simulink model "AbabilFlightController_Android"  (R2021a)
settings: Solver=ode3  StartTime=0.0  StopTime=40.0  RelTol=1e-3
InitFcn:
  | Ts=0.01
  | kFactor = 1.2;
  | 
  | KpRollAttitude = 0.630138625117681 / kFactor;
  | KiRollAttitude = 0.0552303199591522 / kFactor;
  | 
  | KpPitchAttitude = 0.630138625117681 / kFactor;
  | KiPitchAttitude = 0.0552303199591522 / kFactor;
  | 
  | KpRollRate = 1.31533836563383 / kFactor;
  | KiRollRate = 0.460338699849681 / kFactor;
  | 
  | KpPitchRate = 1.31533836563383 / kFactor;
  | KiPitchRate = 0.460338699849681 / kFactor;
  | 
  | KpYawRate = 1.31533836563383 / kFactor;
  | KiYawRate = 0.460338699849681 / kFactor;
undefined symbols (not defined in the file): Accel, AHRS_Ang_Vel, AHRS_Attitude, Alt, androidSerialSendReceive, AttiudeFiltered, Data_Input, fdesignblkfcn, gcbh, Gyro, kalman, Mag, Static_Orientation
libraries: androiduilib x10, androidsensorlib x5, pid_lib x5, androidcommunicationlib x2, mspfiltlib x1, simulink_extras x1, simulink x1, aerolibatmos2 x1
(part 1 of 2)
PreSaveFcn:
  | set_param(gcs, 'Location',[35 56 895 605])
settings Model: ExtModeTrigDuration=100  Creator=The MathWorks, Inc.  LastModifiedBy=AA
settings SolverCC: AlgebraicLoopSolver=TrustRegion
settings DataIOCC: LimitDataPoints=on  SaveFormat=Array  ReturnWorkspaceOutputs=off
settings OptimizationCC: LifeSpan=1  MaxStackSize=64
settings DebuggingCC: UnderspecifiedInitializationDetection=Classic  MergeDetectMultiDrivingBlocksExec=none  ParameterPrecisionLossMsg=none  AllowSymbolicDim=off  SFUnexpectedBacktrackingDiag=warning  SFNoUnconditionalDefaultTransitionDiag=warning  SFExecutionAtInitializationDiag=none  SFMachineParentedDataDiag=warning  ArithmeticOperatorsInVariantConditions=warning
settings HardwareCC: ProdBitPerPointer=32  ProdBitPerSizeT=32  ProdBitPerPtrDiffT=32  ProdLargestAtomicInteger=Long  ProdLargestAtomicFloat=Double  ProdWordSize=32  ProdHWDeviceType=ARM Compatible->ARM Cortex  TargetLargestAtomicInteger=Long  TargetLargestAtomicFloat=Double  TargetEndianess=LittleEndian  TargetHWDeviceType=ARM Compatible->ARM Cortex  UseEmbeddedCoderFeatures=off  UseSimulinkCoderFeatures=off
settings ModelReferenceCC: PropagateSignalLabelsOutOfModel=off
settings SFSimCC: SimUseLocalCustomCode=off  CustomCodeUndefinedFunction=UseInterfaceOnly
settings RTWCC: SystemTargetFile=ert.tlc  HardwareBoard=Android Device  TemplateMakefile=ert_default_tmf  GenerateReport=on  RTWVerbose=off  RTWUseLocalCustomCode=off  Toolchain=Android SDK/NDK Tools  LaunchReport=on
settings CodeAppCC: ForceParamTrailComments=on  OperatorAnnotations=on  StateflowObjectComments=on  MATLABSourceComments=on
settings ERTTargetCC: MultiwordLength=2048  ERTCustomFileBanners=off  SupportContinuousTime=on  SupportNonInlinedSFcns=on  RemoveResetFunc=off  ModelStepFunctionPrototypeControlCompliant=off
settings ConfigComp: CovMetricSettings=dw  CovSaveCumulativeToWorkspaceVar=on  CovSaveSingleToWorkspaceVar=on  CovExternalEMLEnable=off  CovSFcnEnable=off

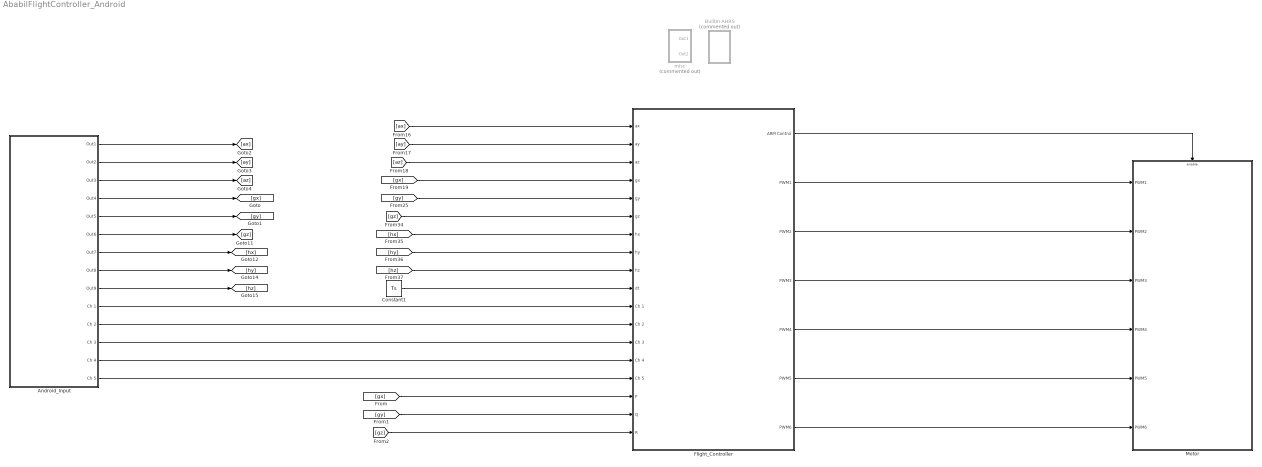
== system AbabilFlightController_Android ==
  Android_Input : Subsystem
  BuiltIn AHRS : Subsystem  Commented=on
  Constant1 : Constant  Value=Ts
  Flight_Controller : Subsystem
  Motor : Subsystem  TreatAsAtomicUnit=on
  misc : Subsystem  Commented=on
  wires:
  Android_Input/3(Out3) -> [az]
  Android_Input/6(Out6) -> [gz]
  [ax] -> Flight_Controller/1(ax)
  [ay] -> Flight_Controller/2(ay)
  [az] -> Flight_Controller/3(az)
  [gy] -> Flight_Controller/5(gy)
  [gx] -> Flight_Controller/4(gx)
  [gz] -> Flight_Controller/6(gz)
  [hz] -> Flight_Controller/9(hz)
  [hy] -> Flight_Controller/8(hy)
  [hx] -> Flight_Controller/7(hx)
  Constant1/1 -> Flight_Controller/10(dt)
  Android_Input/1(Out1) -> [ax]
  Android_Input/2(Out2) -> [ay]
  Android_Input/4(Out4) -> [gx]
  Android_Input/5(Out5) -> [gy]
  Android_Input/7(Out7) -> [hx]
  Android_Input/8(Out8) -> [hy]
  Android_Input/9(Out9) -> [hz]
  [gy] -> Flight_Controller/17(Q)
  [gx] -> Flight_Controller/16(P)
  [gz] -> Flight_Controller/18(R)
  Android_Input/10(Ch 1) -> Flight_Controller/11(Ch 1)
  Android_Input/11(Ch 2) -> Flight_Controller/12(Ch 2)
  Android_Input/12(Ch 3) -> Flight_Controller/13(Ch 3)
  Android_Input/13(Ch 4) -> Flight_Controller/14(Ch 4)
  Android_Input/14(Ch 5) -> Flight_Controller/15(Ch 5)
  Flight_Controller/2(PWM1) -> Motor/1(PWM1)
  Flight_Controller/3(PWM2) -> Motor/2(PWM2)
  Flight_Controller/4(PWM3) -> Motor/3(PWM3)
  Flight_Controller/5(PWM4) -> Motor/4(PWM4)
  Flight_Controller/6(PWM5) -> Motor/5(PWM5)
  Flight_Controller/7(PWM6) -> Motor/6(PWM6)
  Flight_Controller/1(ARM Control) -> Motor/Enable

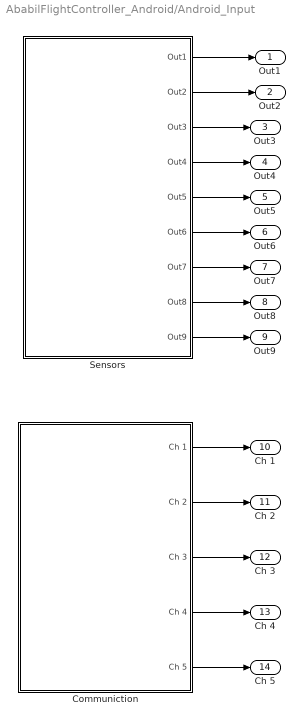
== system AbabilFlightController_Android/Android_Input ==
  Communiction : Subsystem
  Sensors : Subsystem
  Out1 : Outport
  Out2 : Outport  Port=2
  Out3 : Outport  Port=3
  Out4 : Outport  Port=4
  Out5 : Outport  Port=5
  Out6 : Outport  Port=6
  Out7 : Outport  Port=7
  Out8 : Outport  Port=8
  Out9 : Outport  Port=9
  Ch 1 : Outport  Port=10
  Ch 2 : Outport  Port=11
  Ch 3 : Outport  Port=12
  Ch 4 : Outport  Port=13
  Ch 5 : Outport  Port=14
  wires:
  Sensors/1(Out1) -> Out1/1
  Sensors/2(Out2) -> Out2/1
  Sensors/3(Out3) -> Out3/1
  Sensors/4(Out4) -> Out4/1
  Sensors/5(Out5) -> Out5/1
  Sensors/6(Out6) -> Out6/1
  Sensors/7(Out7) -> Out7/1
  Sensors/8(Out8) -> Out8/1
  Sensors/9(Out9) -> Out9/1
  Communiction/1(Ch 1) -> Ch 1/1
  Communiction/2(Ch 2) -> Ch 2/1
  Communiction/3(Ch 3) -> Ch 3/1
  Communiction/4(Ch 4) -> Ch 4/1
  Communiction/5(Ch 5) -> Ch 5/1

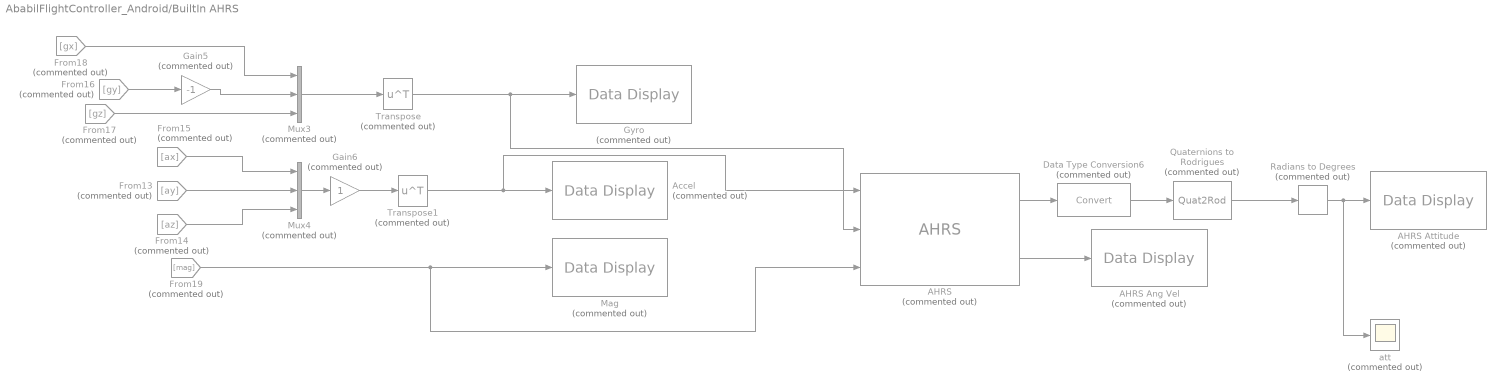
== system AbabilFlightController_Android/BuiltIn AHRS ==
  AHRS : mspfiltlib/AHRS  Commented=on  DispRefFrame=NED  DecimationFactor=1  InitialProcessNoise=ahrsfilter.defaultProcessNoise  OrientationFormat=quaternion  SimulateUsing=Code generation  AccelerometerNoise=7.7792e-07  GyroscopeNoise=3.7046e-08  MagnetometerNoise=0.1  GyroscopeDriftNoise=3.0462e-13  LinearAccelerationNoise=0.0096236100000000012  MagneticDisturbanceNoise=0.5  LinearAccelerationDecayFactor=0.5  MagneticDisturbanceDecayFactor=0.5  ExpectedMagneticFieldStrength=50
      settings: SourceProductBaseCode=TF,NV
  AHRS Ang Vel : androiduilib/Data Display  Commented=on  DataDisplayId=kalman/AHRS_Ang_Vel  Format=Float  Precision=6  SimulateUsing=Code generation  blockPlatform=Android
      settings: SourceProductBaseCode=ANDROID
  AHRS Attitude : androiduilib/Data Display  Commented=on  DataDisplayId=kalman/AHRS_Attitude  Format=Float  Precision=6  SimulateUsing=Code generation  blockPlatform=Android
      settings: SourceProductBaseCode=ANDROID
  Accel : androiduilib/Data Display  Commented=on  DataDisplayId=kalman/Accel  Format=Float  Precision=6  SimulateUsing=Code generation  blockPlatform=Android
      settings: SourceProductBaseCode=ANDROID
  Data Type Conversion6 : DataTypeConversion  Commented=on
  From13 : From  Commented=on  GotoTag=ay
  From14 : From  Commented=on  GotoTag=az
  From15 : From  Commented=on  GotoTag=ax
  From16 : From  Commented=on  GotoTag=gy
  From17 : From  Commented=on  GotoTag=gz
  From18 : From  Commented=on  GotoTag=gx
  From19 : From  Commented=on  GotoTag=mag
  Gain5 : Gain  Commented=on  Gain=-1
  Gain6 : Gain  Commented=on
  Gyro : androiduilib/Data Display  Commented=on  DataDisplayId=kalman/Gyro  Format=Float  Precision=6  SimulateUsing=Code generation  blockPlatform=Android
      settings: SourceProductBaseCode=ANDROID
  Mag : androiduilib/Data Display  Commented=on  DataDisplayId=kalman/Mag  Format=Float  Precision=6  SimulateUsing=Code generation  blockPlatform=Android
      settings: SourceProductBaseCode=ANDROID
  Mux3 : Mux  Commented=on  Inputs=3
  Mux4 : Mux  Commented=on  Inputs=3
  Quaternions to Rodrigues : Quat2Rod  Commented=on
  Radians to Degrees : simulink_extras/Transformations/Radians to Degrees  Commented=on
  Transpose : Math  Commented=on  Operator=transpose  SaturateOnIntegerOverflow=on
  Transpose1 : Math  Commented=on  Operator=transpose  SaturateOnIntegerOverflow=on
  att : Scope  Commented=on
  wires:
  From18/1 -> Mux3/1
  From14/1 -> Mux4/3
  AHRS/2 -> AHRS Ang Vel/1
  Transpose/1 -> AHRS/2, Gyro/1
  From17/1 -> Mux3/3
  Mux4/1 -> Gain6/1
  Transpose1/1 -> AHRS/1, Accel/1
  From15/1 -> Mux4/1
  From19/1 -> AHRS/3, Mag/1
  From13/1 -> Mux4/2
  AHRS/1 -> Data Type Conversion6/1
  Data Type Conversion6/1 -> Quaternions to Rodrigues/1
  Quaternions to Rodrigues/1 -> Radians to Degrees/1
  Radians to Degrees/1 -> att/1, AHRS Attitude/1
  Gain6/1 -> Transpose1/1
  Gain5/1 -> Mux3/2
  From16/1 -> Gain5/1
  Mux3/1 -> Transpose/1

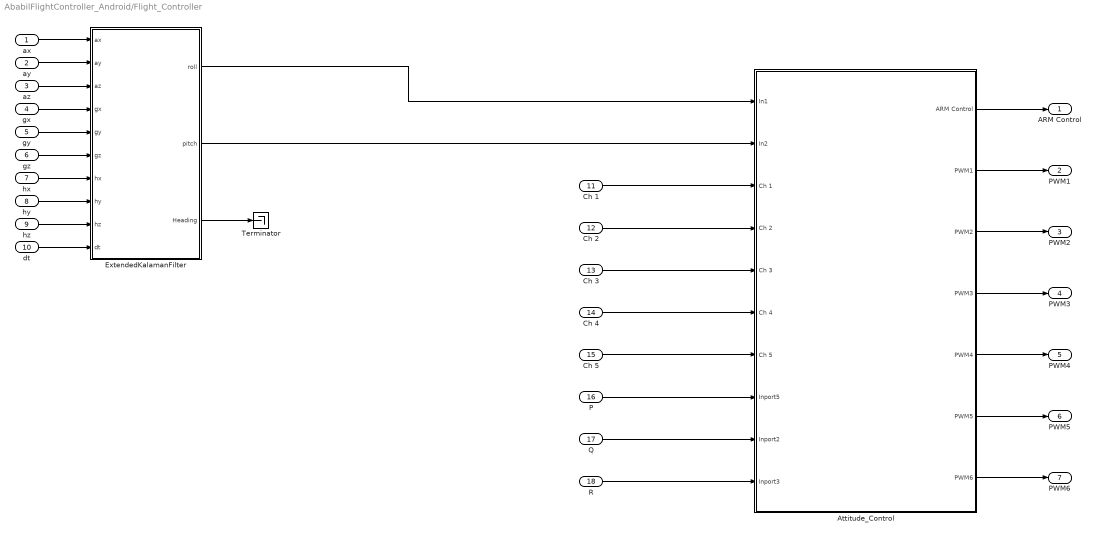
== system AbabilFlightController_Android/Flight_Controller ==
  ax : Inport
  ay : Inport  Port=2
  az : Inport  Port=3
  gx : Inport  Port=4
  gy : Inport  Port=5
  gz : Inport  Port=6
  hx : Inport  Port=7
  hy : Inport  Port=8
  hz : Inport  Port=9
  dt : Inport  Port=10
  Ch 1 : Inport  Port=11
  Ch 2 : Inport  Port=12
  Ch 3 : Inport  Port=13
  Ch 4 : Inport  Port=14
  Ch 5 : Inport  Port=15
  P : Inport  Port=16
  Q : Inport  Port=17
  R : Inport  Port=18
  Attitude_Control : Subsystem
  ExtendedKalamanFilter : Subsystem
  Terminator : Terminator
  ARM Control : Outport
  PWM1 : Outport  Port=2
  PWM2 : Outport  Port=3
  PWM3 : Outport  Port=4
  PWM4 : Outport  Port=5
  PWM5 : Outport  Port=6
  PWM6 : Outport  Port=7
  wires:
  ExtendedKalamanFilter/2(pitch) -> Attitude_Control/2(In2)
  ExtendedKalamanFilter/1(roll) -> Attitude_Control/1(In1)
  ExtendedKalamanFilter/3(Heading) -> Terminator/1
  ax/1 -> ExtendedKalamanFilter/1(ax)
  ay/1 -> ExtendedKalamanFilter/2(ay)
  az/1 -> ExtendedKalamanFilter/3(az)
  gx/1 -> ExtendedKalamanFilter/4(gx)
  gy/1 -> ExtendedKalamanFilter/5(gy)
  gz/1 -> ExtendedKalamanFilter/6(gz)
  hx/1 -> ExtendedKalamanFilter/7(hx)
  hy/1 -> ExtendedKalamanFilter/8(hy)
  hz/1 -> ExtendedKalamanFilter/9(hz)
  dt/1 -> ExtendedKalamanFilter/10(dt)
  Attitude_Control/7(PWM6) -> PWM6/1
  Attitude_Control/6(PWM5) -> PWM5/1
  Attitude_Control/5(PWM4) -> PWM4/1
  Attitude_Control/4(PWM3) -> PWM3/1
  Attitude_Control/3(PWM2) -> PWM2/1
  Attitude_Control/2(PWM1) -> PWM1/1
  Attitude_Control/1(ARM Control) -> ARM Control/1
  Ch 1/1 -> Attitude_Control/3(Ch 1)
  Ch 2/1 -> Attitude_Control/4(Ch 2)
  Ch 3/1 -> Attitude_Control/5(Ch 3)
  Ch 4/1 -> Attitude_Control/6(Ch 4)
  Ch 5/1 -> Attitude_Control/7(Ch 5)
  P/1 -> Attitude_Control/8(Inport5)
  Q/1 -> Attitude_Control/9(Inport2)
  R/1 -> Attitude_Control/10(Inport3)

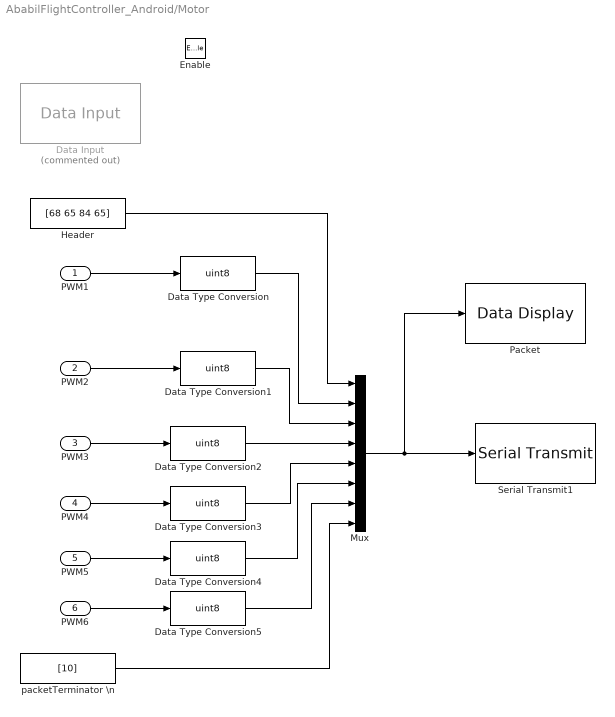
== system AbabilFlightController_Android/Motor ==
  PWM1 : Inport
  PWM2 : Inport  Port=2
  PWM3 : Inport  Port=3
  PWM4 : Inport  Port=4
  PWM5 : Inport  Port=5
  PWM6 : Inport  Port=6
  Enable : EnablePort
  Data Input : androiduilib/Data Input  Commented=on  isCharVector=on  Value=1.0  CharVector=DATA  OutputDataType=double  maxCharVectorSize=4  DataInputId=androidSerialSendReceive/Data_Input  SampleTime=Ts
      settings: SourceProductBaseCode=ANDROID
  Data Type Conversion{,1..5} (6 alike) : DataTypeConversion  OutDataTypeStr=uint8
  Header : Constant  Value=[68 65 84 65]  OutDataTypeStr=uint8  SampleTime=Ts
  Mux : Mux  Inputs=8
  Packet : androiduilib/Data Display  DataDisplayId=Ababil/Motor/Packet  Format=Integer  Precision=6  SimulateUsing=Code generation  blockPlatform=Android
      settings: SourceProductBaseCode=ANDROID
  Serial Transmit1 : androidcommunicationlib/Serial Transmit
      settings: SourceProductBaseCode=ANDROID
  packetTerminator \n : Constant  Value=[10]  OutDataTypeStr=uint8
  wires:
  PWM1/1 -> Data Type Conversion/1
  PWM5/1 -> Data Type Conversion4/1
  PWM2/1 -> Data Type Conversion1/1
  PWM6/1 -> Data Type Conversion5/1
  PWM4/1 -> Data Type Conversion3/1
  Data Type Conversion2/1 -> Mux/4
  Data Type Conversion3/1 -> Mux/5
  Data Type Conversion/1 -> Mux/2
  PWM3/1 -> Data Type Conversion2/1
  Data Type Conversion4/1 -> Mux/6
  Mux/1 -> Packet/1, Serial Transmit1/1
  Data Type Conversion5/1 -> Mux/7
  packetTerminator \n/1 -> Mux/8
  Header/1 -> Mux/1
  Data Type Conversion1/1 -> Mux/3

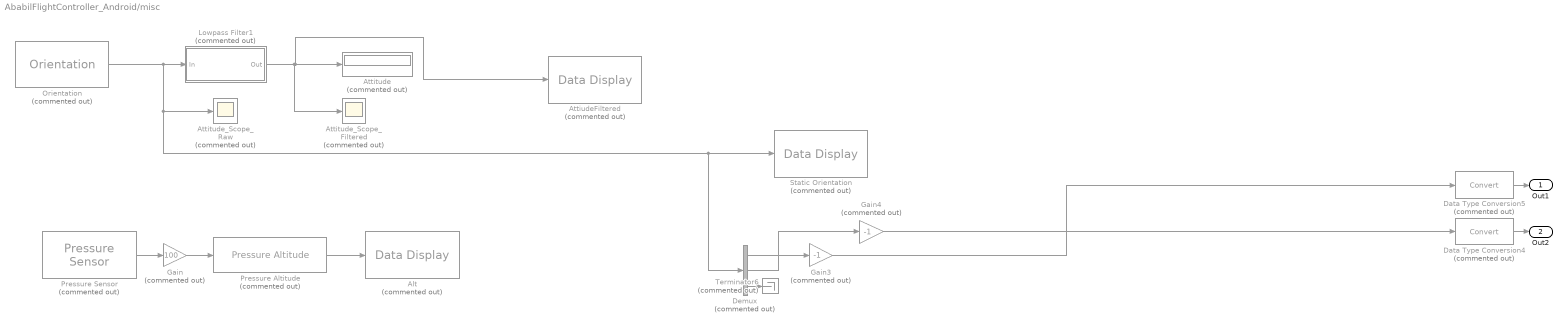
== system AbabilFlightController_Android/misc ==
  Alt : androiduilib/Data Display  Commented=on  DataDisplayId=kalman/Alt  Format=Float  Precision=6  SimulateUsing=Code generation  blockPlatform=Android
      settings: SourceProductBaseCode=ANDROID
  Attitude : Display  Commented=on
  Attitude_Scope_Filtered : Scope  Commented=on
  Attitude_Scope_Raw : Scope  Commented=on
  AttiudeFiltered : androiduilib/Data Display  Commented=on  DataDisplayId=kalman/AttiudeFiltered  Format=Float  Precision=6  SimulateUsing=Code generation  blockPlatform=Android
      settings: SourceProductBaseCode=ANDROID
  Data Type Conversion4 : DataTypeConversion  Commented=on
  Data Type Conversion5 : DataTypeConversion  Commented=on
  Demux : Demux  Commented=on  Outputs=3
  Gain : Gain  Commented=on  Gain=100
  Gain3 : Gain  Commented=on  Gain=-1
  Gain4 : Gain  Commented=on  Gain=-1
  Lowpass Filter1 : Subsystem  Commented=on  DialogController=fdesignblkfcn  InitFcn=fdesignblkfcn(gcbh, {'InitFcn'});  mask(Lowpass Filter){}
      mask help: Design a lowpass filter
      settings: CopyFcn=fdesignblkfcn(gcbh, {'CopyFcn'});
      mask Help: helpview(mapfilelocation('dsp'), 'dsplowpassfilter');
      mask Display: disp('Lowpass')
  Orientation : androidsensorlib/Orientation  Commented=on  SampleTime=Ts
      settings: SourceProductBaseCode=ANDROID
  Pressure Altitude : aerolibatmos2/Pressure Altitude  Commented=on  units=Metric (MKS)  action=Warning
      settings: SourceProductBaseCode=AE
  Pressure Sensor : androidsensorlib/Pressure Sensor  Commented=on  SampleTime=1  BlockPlatform=Android
      settings: SourceProductBaseCode=ANDROID
  Static Orientation : androiduilib/Data Display  Commented=on  DataDisplayId=kalman/Static_Orientation  Format=Float  Precision=6  SimulateUsing=Code generation  blockPlatform=Android
      settings: SourceProductBaseCode=ANDROID
  Terminator6 : Terminator  Commented=on
  Out1 : Outport
  Out2 : Outport  Port=2
  wires:
  Data Type Conversion4/1 -> Out2/1
  Lowpass Filter1/1(Out) -> Attitude_Scope_Filtered/1, AttiudeFiltered/1, Attitude/1
  Gain/1 -> Pressure Altitude/1
  Pressure Sensor/1 -> Gain/1
  Demux/2 -> Gain4/1
  Gain3/1 -> Data Type Conversion5/1
  Orientation/1 -> Attitude_Scope_Raw/1, Demux/1, Static Orientation/1, Lowpass Filter1/1(In)
  Data Type Conversion5/1 -> Out1/1
  Demux/1 -> Gain3/1
  Pressure Altitude/1 -> Alt/1
  Demux/3 -> Terminator6/1
  Gain4/1 -> Data Type Conversion4/1

== system AbabilFlightController_Android/Android_Input/Communiction ==
  BLE Receive : androidcommunicationlib/BLE Receive  DeviceMode=Central (Client)  BluetoothAddress=""  CharUUID=""  ServiceUUID=""  device=No devices  character=No Characteristics  CustomService=off  ServiceName=Heart Rate  CharacteristicName="Heart Rate  Measurement"  CustomServiceUUID=<Enter Service UUID>  CustomCharUUID=<Enter Characteristic UUID>  DataSize=5  SampleTime=Ts  charseruuid=<empty>  seruuid=00001810-0000-1000-8000-00805f9b34fb  PeripheralService=0000180d-0000-1000-8000-00805f9b34fb  PeripheralCharacteristic=00002a37-0000-1000-8000-00805f9b34fb  chruuid=00002a37-0000-1000-8000-00805f9b34fb  BLEId=Ababil/Android_Input/Communiction/BLE_Receive  Devicename=""  IsCustomService=0
      settings: SourceProductBaseCode=ANDROID
  Data Type Conversion{,1..4} (5 alike) : DataTypeConversion  OutDataTypeStr=uint16  RndMeth=Round
  Demux : Demux  Outputs=5
  Terminator : Terminator  Commented=on
  Ch 1 : Outport
  Ch 2 : Outport  Port=2
  Ch 3 : Outport  Port=3
  Ch 4 : Outport  Port=4
  Ch 5 : Outport  Port=5
  wires:
  BLE Receive/2 -> Terminator/1
  Demux/1 -> Data Type Conversion/1
  Data Type Conversion/1 -> Ch 1/1
  Demux/2 -> Data Type Conversion1/1
  Data Type Conversion1/1 -> Ch 2/1
  Demux/3 -> Data Type Conversion2/1
  Data Type Conversion2/1 -> Ch 3/1
  Demux/4 -> Data Type Conversion3/1
  Data Type Conversion3/1 -> Ch 4/1
  Demux/5 -> Data Type Conversion4/1
  Data Type Conversion4/1 -> Ch 5/1
  BLE Receive/1 -> Demux/1

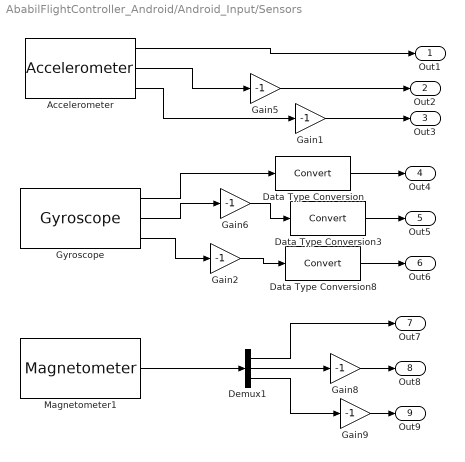
== system AbabilFlightController_Android/Android_Input/Sensors ==
  Accelerometer : androidsensorlib/Accelerometer  OutputVector=off  SampleTime=Ts  BlockPlatform=Android
      settings: SourceProductBaseCode=ANDROID
  Data Type Conversion : DataTypeConversion
  Data Type Conversion3 : DataTypeConversion
  Data Type Conversion8 : DataTypeConversion
  Demux1 : Demux  Outputs=3
  Gain{1..2,5..6,8..9} (6 alike) : Gain  Gain=-1
  Gyroscope : androidsensorlib/Gyroscope  OutputVector=off  SampleTime=Ts  BlockPlatform=Android
      settings: SourceProductBaseCode=ANDROID
  Magnetometer1 : androidsensorlib/Magnetometer  SampleTime=Ts
      settings: SourceProductBaseCode=ANDROID
  Out1 : Outport
  Out2 : Outport  Port=2
  Out3 : Outport  Port=3
  Out4 : Outport  Port=4
  Out5 : Outport  Port=5
  Out6 : Outport  Port=6
  Out7 : Outport  Port=7
  Out8 : Outport  Port=8
  Out9 : Outport  Port=9
  wires:
  Gain5/1 -> Out2/1
  Gain1/1 -> Out3/1
  Data Type Conversion/1 -> Out4/1
  Data Type Conversion3/1 -> Out5/1
  Gain6/1 -> Data Type Conversion3/1
  Gain2/1 -> Data Type Conversion8/1
  Data Type Conversion8/1 -> Out6/1
  Gain8/1 -> Out8/1
  Gain9/1 -> Out9/1
  Magnetometer1/1 -> Demux1/1
  Accelerometer/1 -> Out1/1
  Accelerometer/2 -> Gain5/1
  Accelerometer/3 -> Gain1/1
  Gyroscope/1 -> Data Type Conversion/1
  Gyroscope/2 -> Gain6/1
  Gyroscope/3 -> Gain2/1
  Demux1/1 -> Out7/1
  Demux1/2 -> Gain8/1
  Demux1/3 -> Gain9/1

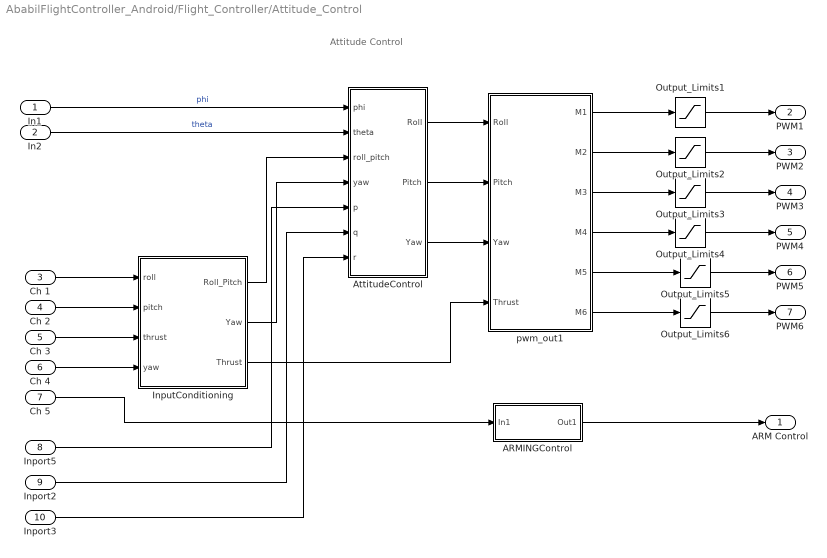
== system AbabilFlightController_Android/Flight_Controller/Attitude_Control ==
  note: Attitude Control
  In1 : Inport
  In2 : Inport  Port=2
  Ch 1 : Inport  Port=3  OutDataTypeStr=uint16
  Ch 2 : Inport  Port=4  OutDataTypeStr=uint16
  Ch 3 : Inport  Port=5  OutDataTypeStr=uint16
  Ch 4 : Inport  Port=6  OutDataTypeStr=uint16
  Ch 5 : Inport  Port=7  OutDataTypeStr=uint16
  Inport5 : Inport  Port=8
  Inport2 : Inport  Port=9
  Inport3 : Inport  Port=10
  ARMINGControl : Subsystem
  AttitudeControl : Subsystem
  InputConditioning : Subsystem
  Output_Limits{1..6} (6 alike) : Saturate  UpperLimit=200  LowerLimit=100
  pwm_out1 : MATLAB Function  TreatAsAtomicUnit=on  SystemSampleTime=0.004
  ARM Control : Outport
  PWM1 : Outport  Port=2
  PWM2 : Outport  Port=3
  PWM3 : Outport  Port=4
  PWM4 : Outport  Port=5
  PWM5 : Outport  Port=6
  PWM6 : Outport  Port=7
  wires:
  AttitudeControl/1(Roll) -> pwm_out1/1(Roll)
  Ch 3/1 -> InputConditioning/3(thrust)
  pwm_out1/3(M3) -> Output_Limits3/1
  pwm_out1/5(M5) -> Output_Limits5/1
  AttitudeControl/2(Pitch) -> pwm_out1/2(Pitch)
  Ch 2/1 -> InputConditioning/2(pitch)
  Ch 4/1 -> InputConditioning/4(yaw)
  Output_Limits1/1 -> PWM1/1
  Inport3/1 -> AttitudeControl/7(r)
  In1/1 -> AttitudeControl/1(phi)  "phi"
  ARMINGControl/1(Out1) -> ARM Control/1
  AttitudeControl/3(Yaw) -> pwm_out1/3(Yaw)
  pwm_out1/2(M2) -> Output_Limits2/1
  Ch 1/1 -> InputConditioning/1(roll)
  InputConditioning/3(Thrust) -> pwm_out1/4(Thrust)
  Inport2/1 -> AttitudeControl/6(q)
  pwm_out1/1(M1) -> Output_Limits1/1
  pwm_out1/4(M4) -> Output_Limits4/1
  InputConditioning/1(Roll_Pitch) -> AttitudeControl/3(roll_pitch)
  InputConditioning/2(Yaw) -> AttitudeControl/4(yaw)
  pwm_out1/6(M6) -> Output_Limits6/1
  Ch 5/1 -> ARMINGControl/1(In1)
  Inport5/1 -> AttitudeControl/5(p)
  In2/1 -> AttitudeControl/2(theta)  "theta"
  Output_Limits2/1 -> PWM2/1
  Output_Limits3/1 -> PWM3/1
  Output_Limits4/1 -> PWM4/1
  Output_Limits5/1 -> PWM5/1
  Output_Limits6/1 -> PWM6/1

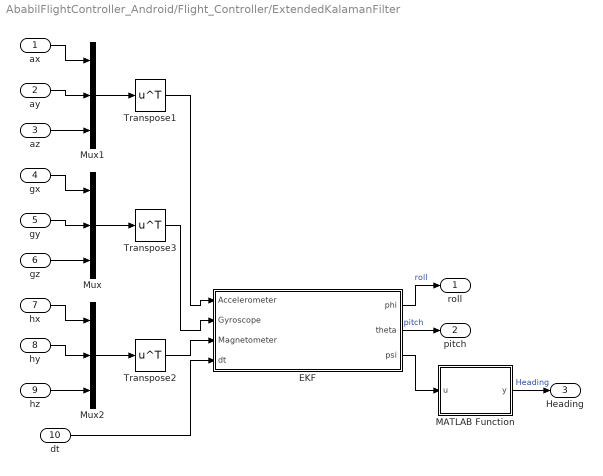
== system AbabilFlightController_Android/Flight_Controller/ExtendedKalamanFilter ==
  ax : Inport
  ay : Inport  Port=2
  az : Inport  Port=3
  gx : Inport  Port=4
  gy : Inport  Port=5
  gz : Inport  Port=6
  hx : Inport  Port=7
  hy : Inport  Port=8
  hz : Inport  Port=9
  dt : Inport  Port=10
  EKF : MATLAB Function  TreatAsAtomicUnit=on
  MATLAB Function : MATLAB Function  TreatAsAtomicUnit=on
  Mux : Mux  Inputs=3
  Mux1 : Mux  Inputs=3
  Mux2 : Mux  Inputs=3
  Transpose1 : Math  Operator=transpose  SaturateOnIntegerOverflow=on
  Transpose2 : Math  Operator=transpose  SaturateOnIntegerOverflow=on
  Transpose3 : Math  Operator=transpose  SaturateOnIntegerOverflow=on
  roll : Outport
  pitch : Outport  Port=2
  Heading : Outport  Port=3
  wires:
  MATLAB Function/1(y) -> Heading/1  "Heading"
  gy/1 -> Mux/2
  gz/1 -> Mux/3
  hz/1 -> Mux2/3
  ax/1 -> Mux1/1
  az/1 -> Mux1/3
  EKF/1(phi) -> roll/1  "roll"
  ay/1 -> Mux1/2
  Mux2/1 -> Transpose2/1
  Transpose1/1 -> EKF/1(Accelerometer)
  hx/1 -> Mux2/1
  Transpose2/1 -> EKF/3(Magnetometer)
  Mux1/1 -> Transpose1/1
  Mux/1 -> Transpose3/1
  EKF/3(psi) -> MATLAB Function/1(u)
  EKF/2(theta) -> pitch/1  "pitch"
  gx/1 -> Mux/1
  hy/1 -> Mux2/2
  Transpose3/1 -> EKF/2(Gyroscope)
  dt/1 -> EKF/4(dt)

== system AbabilFlightController_Android/misc/Lowpass Filter1 ==
  In : Inport
  Generated Filter Block : Subsystem  Tag=FilterWizardSubSystem
      settings: ErrorFcn=dspFilterRealizedInBasicElemsAlgLoopErrFcnCallback
  Out : Outport
  wires:
  In/1 -> Generated Filter Block/1(Input)
  Generated Filter Block/1(Output) -> Out/1

== system AbabilFlightController_Android/Flight_Controller/Attitude_Control/ARMINGControl ==
  In1 : Inport
  Compare To Constant3 : simulink/Logic and Bit Operations/Compare To Constant  relop=>=  const=150  OutDataTypeStr=boolean
  Out1 : Outport  VectorParamsAs1DForOutWhenUnconnected=off
  wires:
  Compare To Constant3/1 -> Out1/1
  In1/1 -> Compare To Constant3/1

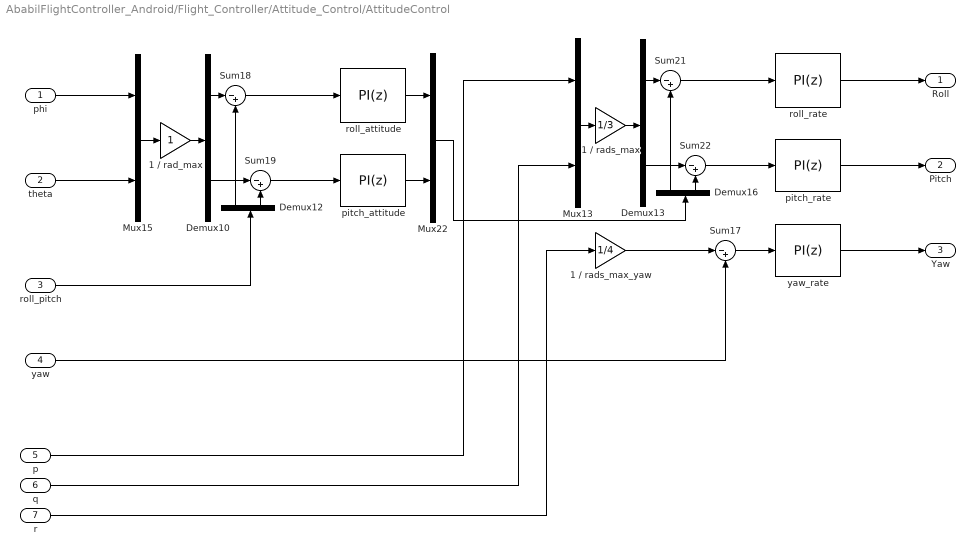
== system AbabilFlightController_Android/Flight_Controller/Attitude_Control/AttitudeControl ==
  phi : Inport
  theta : Inport  Port=2
  roll_pitch : Inport  Port=3
  yaw : Inport  Port=4
  p : Inport  Port=5
  q : Inport  Port=6
  r : Inport  Port=7
  1 / rad_max : Gain
  1 / rads_max : Gain  Gain=1/3
  1 / rads_max_yaw : Gain  Gain=1/4
  Demux{10,12..13,16} (4 alike) : Demux  Outputs=2
  Mux13 : Mux  Inputs=2
  Mux15 : Mux  Inputs=2
  Mux22 : Mux  Inputs=2
  Sum{17..19,21..22} (5 alike) : Sum  Inputs=|-+
  pitch_attitude : pid_lib/PID Controller  Controller=PI  Form=Parallel  TimeDomain=Discrete-time  UseExternalTs=off  SampleTime=-1  IntegratorMethod=Forward Euler  FilterMethod=Forward Euler  ControllerParametersSource=internal  P=KpPitchAttitude  I=KiPitchAttitude  D=0.01  UseFilter=on  N=100  TunerSelectOption=Transfer Function Based (PID Tuner App)  InitialConditionSource=internal  InitialConditionForIntegrator=0  InitialConditionForFilter=0  DifferentiatorICPrevScaledInput=0  ExternalReset=none  TrackingMode=off  Kt=1  LimitOutput=on  SatLimitsSource=internal  UpperSaturationLimit=1  LowerSaturationLimit=-1  LinearizeAsGain=on  AntiWindupMode=back-calculation  Kb=1  POutMin=[]  POutMax=[]  IOutMin=[]  IOutMax=[]  DOutMin=[]  DOutMax=[]  NOutMin=[]  NOutMax=[]  SumOutMin=[]  SumOutMax=[]  SaturationOutMin=[]  SaturationOutMax=[]  PParamMin=[]  PParamMax=[]  IParamMin=[]  IParamMax=[]  DParamMin=[]  DParamMax=[]  NParamMin=[]  NParamMax=[]  KbParamMin=[]  KbParamMax=[]  KtParamMin=[]  KtParamMax=[]  KbOutMin=[]  KbOutMax=[]  KtOutMin=[]  KtOutMax=[]  IntegratorOutMin=[]  IntegratorOutMax=[]  FilterOutMin=[]  FilterOutMax=[]  SumI1OutMin=[]  SumI1OutMax=[]  SumI2OutMin=[]  SumI2OutMax=[]  SumI3OutMin=[]  SumI3OutMax=[]  SumI4OutMin=[]  SumI4OutMax=[]  SumDOutMin=[]  SumDOutMax=[]  DifferentiatorOutMin=[]  DifferentiatorOutMax=[]  FilterDiffOutCoefMin=[]  FilterDiffOutCoefMax=[]  ReciprocalOutMin=[]  ReciprocalOutMax=[]  SumDenOutMin=[]  SumDenOutMax=[]  SumNumOutMin=[]  SumNumOutMax=[]  DivideOutMin=[]  DivideOutMax=[]  UdiffTsProdOutMin=[]  UdiffTsProdOutMax=[]  NTsProdOutMin=[]  NTsProdOutMax=[]  UintegralTsProdOutMin=[]  UintegralTsProdOutMax=[]  UngainTsProdOutMin=[]  UngainTsProdOutMax=[]  IntegratorContinuousStateAttributes=''  IntegratorStateMustResolveToSignalObject=off  IntegratorRTWStateStorageClass=Auto  FilterContinuousStateAttributes=''  FilterStateMustResolveToSignalObject=off  FilterRTWStateStorageClass=Auto  ParallelPVariant=InternalParameters  IdealPVariant=Disabled  IVariant=InternalParameters  DVariant=Disabled  IntegratorVariant=Discrete  SatVariant=Enabled  AWVariant=BackCalculation  PCopyVariant=Disabled  TRVariant=Disabled  FdbkBlocksVariant=Forward  IdealPFdbkVariant=Disabled  SatFdbkVariant=Disabled  DerivativeFilterVariant=Disabled  NVariant=Disabled  NCopyVariant=Disabled_SignalSpec  FilterICVariant=Disabled  IntegratorICVariant=InternalICs  ExternalResetVariant=Disabled  TRSumVariant=Passthrough  SumFdbkVariant=Disabled  SumVariant=Sum_PI  TsampFilterVariant=InternalTs  TsampNgainVariant=Passthrough  TsampIntegralVariant=Passthrough  ExternalSaturationOutDataTypeStr=Inherit: Same as second input
  pitch_rate : pid_lib/PID Controller  Controller=PI  Form=Parallel  TimeDomain=Discrete-time  UseExternalTs=off  SampleTime=-1  IntegratorMethod=Forward Euler  FilterMethod=Forward Euler  ControllerParametersSource=internal  P=KpPitchRate  I=KiPitchRate  D=0.0024  UseFilter=on  N=100  TunerSelectOption=Transfer Function Based (PID Tuner App)  InitialConditionSource=internal  InitialConditionForIntegrator=0  InitialConditionForFilter=0  DifferentiatorICPrevScaledInput=0  ExternalReset=none  TrackingMode=off  Kt=1  LimitOutput=on  SatLimitsSource=internal  UpperSaturationLimit=1  LowerSaturationLimit=-1  LinearizeAsGain=on  AntiWindupMode=back-calculation  Kb=1  POutMin=[]  POutMax=[]  IOutMin=[]  IOutMax=[]  DOutMin=[]  DOutMax=[]  NOutMin=[]  NOutMax=[]  SumOutMin=[]  SumOutMax=[]  SaturationOutMin=[]  SaturationOutMax=[]  PParamMin=[]  PParamMax=[]  IParamMin=[]  IParamMax=[]  DParamMin=[]  DParamMax=[]  NParamMin=[]  NParamMax=[]  KbParamMin=[]  KbParamMax=[]  KtParamMin=[]  KtParamMax=[]  KbOutMin=[]  KbOutMax=[]  KtOutMin=[]  KtOutMax=[]  IntegratorOutMin=[]  IntegratorOutMax=[]  FilterOutMin=[]  FilterOutMax=[]  SumI1OutMin=[]  SumI1OutMax=[]  SumI2OutMin=[]  SumI2OutMax=[]  SumI3OutMin=[]  SumI3OutMax=[]  SumI4OutMin=[]  SumI4OutMax=[]  SumDOutMin=[]  SumDOutMax=[]  DifferentiatorOutMin=[]  DifferentiatorOutMax=[]  FilterDiffOutCoefMin=[]  FilterDiffOutCoefMax=[]  ReciprocalOutMin=[]  ReciprocalOutMax=[]  SumDenOutMin=[]  SumDenOutMax=[]  SumNumOutMin=[]  SumNumOutMax=[]  DivideOutMin=[]  DivideOutMax=[]  UdiffTsProdOutMin=[]  UdiffTsProdOutMax=[]  NTsProdOutMin=[]  NTsProdOutMax=[]  UintegralTsProdOutMin=[]  UintegralTsProdOutMax=[]  UngainTsProdOutMin=[]  UngainTsProdOutMax=[]  IntegratorContinuousStateAttributes=''  IntegratorStateMustResolveToSignalObject=off  IntegratorRTWStateStorageClass=Auto  FilterContinuousStateAttributes=''  FilterStateMustResolveToSignalObject=off  FilterRTWStateStorageClass=Auto  ParallelPVariant=InternalParameters  IdealPVariant=Disabled  IVariant=InternalParameters  DVariant=Disabled  IntegratorVariant=Discrete  SatVariant=Enabled  AWVariant=BackCalculation  PCopyVariant=Disabled  TRVariant=Disabled  FdbkBlocksVariant=Forward  IdealPFdbkVariant=Disabled  SatFdbkVariant=Disabled  DerivativeFilterVariant=Disabled  NVariant=Disabled  NCopyVariant=Disabled_SignalSpec  FilterICVariant=Disabled  IntegratorICVariant=InternalICs  ExternalResetVariant=Disabled  TRSumVariant=Passthrough  SumFdbkVariant=Disabled  SumVariant=Sum_PI  TsampFilterVariant=InternalTs  TsampNgainVariant=Passthrough  TsampIntegralVariant=Passthrough  ExternalSaturationOutDataTypeStr=Inherit: Same as second input
  roll_attitude : pid_lib/PID Controller  Controller=PI  Form=Parallel  TimeDomain=Discrete-time  UseExternalTs=off  SampleTime=-1  IntegratorMethod=Forward Euler  FilterMethod=Forward Euler  ControllerParametersSource=internal  P=KpRollAttitude  I=KiRollAttitude  D=0.01  UseFilter=on  N=100  TunerSelectOption=Transfer Function Based (PID Tuner App)  InitialConditionSource=internal  InitialConditionForIntegrator=0  InitialConditionForFilter=0  DifferentiatorICPrevScaledInput=0  ExternalReset=none  TrackingMode=off  Kt=1  LimitOutput=on  SatLimitsSource=internal  UpperSaturationLimit=1  LowerSaturationLimit=-1  LinearizeAsGain=on  AntiWindupMode=back-calculation  Kb=1  POutMin=[]  POutMax=[]  IOutMin=[]  IOutMax=[]  DOutMin=[]  DOutMax=[]  NOutMin=[]  NOutMax=[]  SumOutMin=[]  SumOutMax=[]  SaturationOutMin=[]  SaturationOutMax=[]  PParamMin=[]  PParamMax=[]  IParamMin=[]  IParamMax=[]  DParamMin=[]  DParamMax=[]  NParamMin=[]  NParamMax=[]  KbParamMin=[]  KbParamMax=[]  KtParamMin=[]  KtParamMax=[]  KbOutMin=[]  KbOutMax=[]  KtOutMin=[]  KtOutMax=[]  IntegratorOutMin=[]  IntegratorOutMax=[]  FilterOutMin=[]  FilterOutMax=[]  SumI1OutMin=[]  SumI1OutMax=[]  SumI2OutMin=[]  SumI2OutMax=[]  SumI3OutMin=[]  SumI3OutMax=[]  SumI4OutMin=[]  SumI4OutMax=[]  SumDOutMin=[]  SumDOutMax=[]  DifferentiatorOutMin=[]  DifferentiatorOutMax=[]  FilterDiffOutCoefMin=[]  FilterDiffOutCoefMax=[]  ReciprocalOutMin=[]  ReciprocalOutMax=[]  SumDenOutMin=[]  SumDenOutMax=[]  SumNumOutMin=[]  SumNumOutMax=[]  DivideOutMin=[]  DivideOutMax=[]  UdiffTsProdOutMin=[]  UdiffTsProdOutMax=[]  NTsProdOutMin=[]  NTsProdOutMax=[]  UintegralTsProdOutMin=[]  UintegralTsProdOutMax=[]  UngainTsProdOutMin=[]  UngainTsProdOutMax=[]  IntegratorContinuousStateAttributes=''  IntegratorStateMustResolveToSignalObject=off  IntegratorRTWStateStorageClass=Auto  FilterContinuousStateAttributes=''  FilterStateMustResolveToSignalObject=off  FilterRTWStateStorageClass=Auto  ParallelPVariant=InternalParameters  IdealPVariant=Disabled  IVariant=InternalParameters  DVariant=Disabled  IntegratorVariant=Discrete  SatVariant=Enabled  AWVariant=BackCalculation  PCopyVariant=Disabled  TRVariant=Disabled  FdbkBlocksVariant=Forward  IdealPFdbkVariant=Disabled  SatFdbkVariant=Disabled  DerivativeFilterVariant=Disabled  NVariant=Disabled  NCopyVariant=Disabled_SignalSpec  FilterICVariant=Disabled  IntegratorICVariant=InternalICs  ExternalResetVariant=Disabled  TRSumVariant=Passthrough  SumFdbkVariant=Disabled  SumVariant=Sum_PI  TsampFilterVariant=InternalTs  TsampNgainVariant=Passthrough  TsampIntegralVariant=Passthrough  ExternalSaturationOutDataTypeStr=Inherit: Same as second input
  roll_rate : pid_lib/PID Controller  Controller=PI  Form=Parallel  TimeDomain=Discrete-time  UseExternalTs=off  SampleTime=-1  IntegratorMethod=Forward Euler  FilterMethod=Forward Euler  ControllerParametersSource=internal  P=KpRollRate  I=KiRollRate  D=0.0024  UseFilter=on  N=100  TunerSelectOption=Transfer Function Based (PID Tuner App)  InitialConditionSource=internal  InitialConditionForIntegrator=0  InitialConditionForFilter=0  DifferentiatorICPrevScaledInput=0  ExternalReset=none  TrackingMode=off  Kt=1  LimitOutput=on  SatLimitsSource=internal  UpperSaturationLimit=1  LowerSaturationLimit=-1  LinearizeAsGain=on  AntiWindupMode=back-calculation  Kb=1  POutMin=[]  POutMax=[]  IOutMin=[]  IOutMax=[]  DOutMin=[]  DOutMax=[]  NOutMin=[]  NOutMax=[]  SumOutMin=[]  SumOutMax=[]  SaturationOutMin=[]  SaturationOutMax=[]  PParamMin=[]  PParamMax=[]  IParamMin=[]  IParamMax=[]  DParamMin=[]  DParamMax=[]  NParamMin=[]  NParamMax=[]  KbParamMin=[]  KbParamMax=[]  KtParamMin=[]  KtParamMax=[]  KbOutMin=[]  KbOutMax=[]  KtOutMin=[]  KtOutMax=[]  IntegratorOutMin=[]  IntegratorOutMax=[]  FilterOutMin=[]  FilterOutMax=[]  SumI1OutMin=[]  SumI1OutMax=[]  SumI2OutMin=[]  SumI2OutMax=[]  SumI3OutMin=[]  SumI3OutMax=[]  SumI4OutMin=[]  SumI4OutMax=[]  SumDOutMin=[]  SumDOutMax=[]  DifferentiatorOutMin=[]  DifferentiatorOutMax=[]  FilterDiffOutCoefMin=[]  FilterDiffOutCoefMax=[]  ReciprocalOutMin=[]  ReciprocalOutMax=[]  SumDenOutMin=[]  SumDenOutMax=[]  SumNumOutMin=[]  SumNumOutMax=[]  DivideOutMin=[]  DivideOutMax=[]  UdiffTsProdOutMin=[]  UdiffTsProdOutMax=[]  NTsProdOutMin=[]  NTsProdOutMax=[]  UintegralTsProdOutMin=[]  UintegralTsProdOutMax=[]  UngainTsProdOutMin=[]  UngainTsProdOutMax=[]  IntegratorContinuousStateAttributes=''  IntegratorStateMustResolveToSignalObject=off  IntegratorRTWStateStorageClass=Auto  FilterContinuousStateAttributes=''  FilterStateMustResolveToSignalObject=off  FilterRTWStateStorageClass=Auto  ParallelPVariant=InternalParameters  IdealPVariant=Disabled  IVariant=InternalParameters  DVariant=Disabled  IntegratorVariant=Discrete  SatVariant=Enabled  AWVariant=BackCalculation  PCopyVariant=Disabled  TRVariant=Disabled  FdbkBlocksVariant=Forward  IdealPFdbkVariant=Disabled  SatFdbkVariant=Disabled  DerivativeFilterVariant=Disabled  NVariant=Disabled  NCopyVariant=Disabled_SignalSpec  FilterICVariant=Disabled  IntegratorICVariant=InternalICs  ExternalResetVariant=Disabled  TRSumVariant=Passthrough  SumFdbkVariant=Disabled  SumVariant=Sum_PI  TsampFilterVariant=InternalTs  TsampNgainVariant=Passthrough  TsampIntegralVariant=Passthrough  ExternalSaturationOutDataTypeStr=Inherit: Same as second input
  yaw_rate : pid_lib/PID Controller  Controller=PI  Form=Parallel  TimeDomain=Discrete-time  UseExternalTs=off  SampleTime=-1  IntegratorMethod=Forward Euler  FilterMethod=Forward Euler  ControllerParametersSource=internal  P=KpYawRate  I=KiYawRate  D=0  UseFilter=on  N=100  TunerSelectOption=Transfer Function Based (PID Tuner App)  InitialConditionSource=internal  InitialConditionForIntegrator=0  InitialConditionForFilter=0  DifferentiatorICPrevScaledInput=0  ExternalReset=none  TrackingMode=off  Kt=1  LimitOutput=on  SatLimitsSource=internal  UpperSaturationLimit=1  LowerSaturationLimit=-1  LinearizeAsGain=on  AntiWindupMode=back-calculation  Kb=1  POutMin=[]  POutMax=[]  IOutMin=[]  IOutMax=[]  DOutMin=[]  DOutMax=[]  NOutMin=[]  NOutMax=[]  SumOutMin=[]  SumOutMax=[]  SaturationOutMin=[]  SaturationOutMax=[]  PParamMin=[]  PParamMax=[]  IParamMin=[]  IParamMax=[]  DParamMin=[]  DParamMax=[]  NParamMin=[]  NParamMax=[]  KbParamMin=[]  KbParamMax=[]  KtParamMin=[]  KtParamMax=[]  KbOutMin=[]  KbOutMax=[]  KtOutMin=[]  KtOutMax=[]  IntegratorOutMin=[]  IntegratorOutMax=[]  FilterOutMin=[]  FilterOutMax=[]  SumI1OutMin=[]  SumI1OutMax=[]  SumI2OutMin=[]  SumI2OutMax=[]  SumI3OutMin=[]  SumI3OutMax=[]  SumI4OutMin=[]  SumI4OutMax=[]  SumDOutMin=[]  SumDOutMax=[]  DifferentiatorOutMin=[]  DifferentiatorOutMax=[]  FilterDiffOutCoefMin=[]  FilterDiffOutCoefMax=[]  ReciprocalOutMin=[]  ReciprocalOutMax=[]  SumDenOutMin=[]  SumDenOutMax=[]  SumNumOutMin=[]  SumNumOutMax=[]  DivideOutMin=[]  DivideOutMax=[]  UdiffTsProdOutMin=[]  UdiffTsProdOutMax=[]  NTsProdOutMin=[]  NTsProdOutMax=[]  UintegralTsProdOutMin=[]  UintegralTsProdOutMax=[]  UngainTsProdOutMin=[]  UngainTsProdOutMax=[]  IntegratorContinuousStateAttributes=''  IntegratorStateMustResolveToSignalObject=off  IntegratorRTWStateStorageClass=Auto  FilterContinuousStateAttributes=''  FilterStateMustResolveToSignalObject=off  FilterRTWStateStorageClass=Auto  ParallelPVariant=InternalParameters  IdealPVariant=Disabled  IVariant=InternalParameters  DVariant=Disabled  IntegratorVariant=Discrete  SatVariant=Enabled  AWVariant=BackCalculation  PCopyVariant=Disabled  TRVariant=Disabled  FdbkBlocksVariant=Forward  IdealPFdbkVariant=Disabled  SatFdbkVariant=Disabled  DerivativeFilterVariant=Disabled  NVariant=Disabled  NCopyVariant=Disabled_SignalSpec  FilterICVariant=Disabled  IntegratorICVariant=InternalICs  ExternalResetVariant=Disabled  TRSumVariant=Passthrough  SumFdbkVariant=Disabled  SumVariant=Sum_PI  TsampFilterVariant=InternalTs  TsampNgainVariant=Passthrough  TsampIntegralVariant=Passthrough  ExternalSaturationOutDataTypeStr=Inherit: Same as second input
  Roll : Outport  VectorParamsAs1DForOutWhenUnconnected=off
  Pitch : Outport  Port=2  VectorParamsAs1DForOutWhenUnconnected=off
  Yaw : Outport  Port=3  VectorParamsAs1DForOutWhenUnconnected=off
  wires:
  r/1 -> 1 / rads_max_yaw/1
  q/1 -> Mux13/2
  Mux22/1 -> Demux16/1
  yaw_rate/1 -> Yaw/1
  phi/1 -> Mux15/1
  Mux15/1 -> 1 / rad_max/1
  theta/1 -> Mux15/2
  1 / rads_max_yaw/1 -> Sum17/1
  roll_rate/1 -> Roll/1
  Sum19/1 -> pitch_attitude/1
  pitch_attitude/1 -> Mux22/2
  roll_attitude/1 -> Mux22/1
  Demux16/1 -> Sum21/2
  yaw/1 -> Sum17/2
  roll_pitch/1 -> Demux12/1
  Demux16/2 -> Sum22/2
  Demux12/1 -> Sum18/2
  Demux12/2 -> Sum19/2
  p/1 -> Mux13/1
  Demux10/1 -> Sum18/1
  Demux10/2 -> Sum19/1
  1 / rad_max/1 -> Demux10/1
  Sum18/1 -> roll_attitude/1
  pitch_rate/1 -> Pitch/1
  Mux13/1 -> 1 / rads_max/1
  Sum22/1 -> pitch_rate/1
  Sum17/1 -> yaw_rate/1
  Demux13/1 -> Sum21/1
  Demux13/2 -> Sum22/1
  1 / rads_max/1 -> Demux13/1
  Sum21/1 -> roll_rate/1

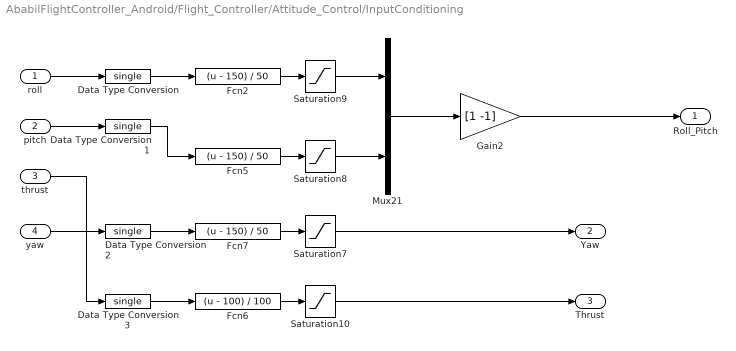
== system AbabilFlightController_Android/Flight_Controller/Attitude_Control/InputConditioning ==
  roll : Inport
  pitch : Inport  Port=2
  thrust : Inport  Port=3
  yaw : Inport  Port=4
  Data Type Conversion{,1..3} (4 alike) : DataTypeConversion  OutDataTypeStr=single
  Fcn2 : Fcn  Expr=(u - 150) / 50
  Fcn5 : Fcn  Expr=(u - 150) / 50
  Fcn6 : Fcn  Expr=(u - 100) / 100
  Fcn7 : Fcn  Expr=(u - 150) / 50
  Gain2 : Gain  Gain=[1 -1]  OutDataTypeStr=Inherit: Inherit via back propagation
  Mux21 : Mux  Inputs=2
  Saturation10 : Saturate  UpperLimit=1  LowerLimit=0
  Saturation7 : Saturate  UpperLimit=1  LowerLimit=-1
  Saturation8 : Saturate  UpperLimit=1  LowerLimit=-1
  Saturation9 : Saturate  UpperLimit=1  LowerLimit=-1
  Roll_Pitch : Outport  VectorParamsAs1DForOutWhenUnconnected=off
  Yaw : Outport  Port=2  VectorParamsAs1DForOutWhenUnconnected=off
  Thrust : Outport  Port=3  VectorParamsAs1DForOutWhenUnconnected=off
  wires:
  Saturation10/1 -> Thrust/1
  Saturation7/1 -> Yaw/1
  Gain2/1 -> Roll_Pitch/1
  Mux21/1 -> Gain2/1
  Saturation8/1 -> Mux21/2
  Fcn6/1 -> Saturation10/1
  thrust/1 -> Data Type Conversion3/1
  Fcn2/1 -> Saturation9/1
  Fcn5/1 -> Saturation8/1
  Saturation9/1 -> Mux21/1
  Fcn7/1 -> Saturation7/1
  yaw/1 -> Data Type Conversion2/1
  pitch/1 -> Data Type Conversion1/1
  roll/1 -> Data Type Conversion/1
  Data Type Conversion/1 -> Fcn2/1
  Data Type Conversion1/1 -> Fcn5/1
  Data Type Conversion2/1 -> Fcn7/1
  Data Type Conversion3/1 -> Fcn6/1

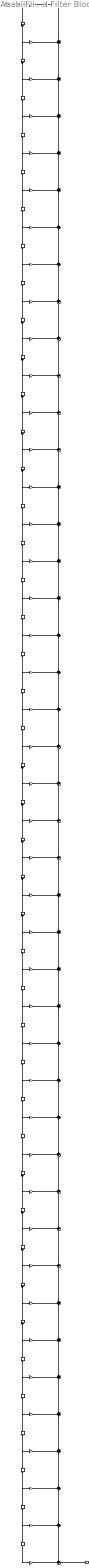
== system AbabilFlightController_Android/misc/Lowpass Filter1/Generated Filter Block ==
  Input : Inport
  BodyDelay{2..43} (42 alike) : Delay  DelayLength=1  InitialCondition=0
  BodyLSum{2..43} (42 alike) : Sum  Inputs=++|  RndMeth=Nearest  SaturateOnIntegerOverflow=on  OutDataTypeStr=Inherit: Same as first input
  b(1) : Gain  Gain=-0.00242287385232693503  ParamDataTypeStr=double  RndMeth=Nearest  SaturateOnIntegerOverflow=on  OutDataTypeStr=Inherit: Same as input
  b(10) : Gain  Gain=-0.0101212347032790025  ParamDataTypeStr=double  RndMeth=Nearest  SaturateOnIntegerOverflow=on  OutDataTypeStr=Inherit: Same as input
  b(11) : Gain  Gain=-0.0182735187337824609  ParamDataTypeStr=double  RndMeth=Nearest  SaturateOnIntegerOverflow=on  OutDataTypeStr=Inherit: Same as input
  b(12) : Gain  Gain=0.0114319620717779676  ParamDataTypeStr=double  RndMeth=Nearest  SaturateOnIntegerOverflow=on  OutDataTypeStr=Inherit: Same as input
  b(13) : Gain  Gain=0.026175888580407581  ParamDataTypeStr=double  RndMeth=Nearest  SaturateOnIntegerOverflow=on  OutDataTypeStr=Inherit: Same as input
  b(14) : Gain  Gain=-0.0124890278353230171  ParamDataTypeStr=double  RndMeth=Nearest  SaturateOnIntegerOverflow=on  OutDataTypeStr=Inherit: Same as input
  b(15) : Gain  Gain=-0.0379966231454636413  ParamDataTypeStr=double  RndMeth=Nearest  SaturateOnIntegerOverflow=on  OutDataTypeStr=Inherit: Same as input
  b(16) : Gain  Gain=0.0133889451993669008  ParamDataTypeStr=double  RndMeth=Nearest  SaturateOnIntegerOverflow=on  OutDataTypeStr=Inherit: Same as input
  b(17) : Gain  Gain=0.0581554658147298703  ParamDataTypeStr=double  RndMeth=Nearest  SaturateOnIntegerOverflow=on  OutDataTypeStr=Inherit: Same as input
  b(18) : Gain  Gain=-0.0140480435158088935  ParamDataTypeStr=double  RndMeth=Nearest  SaturateOnIntegerOverflow=on  OutDataTypeStr=Inherit: Same as input
  b(19) : Gain  Gain=-0.102724668578821676  ParamDataTypeStr=double  RndMeth=Nearest  SaturateOnIntegerOverflow=on  OutDataTypeStr=Inherit: Same as input
  b(2) : Gain  Gain=-0.00208324498207925878  ParamDataTypeStr=double  RndMeth=Nearest  SaturateOnIntegerOverflow=on  OutDataTypeStr=Inherit: Same as input
  b(20) : Gain  Gain=0.0144622757712384552  ParamDataTypeStr=double  RndMeth=Nearest  SaturateOnIntegerOverflow=on  OutDataTypeStr=Inherit: Same as input
  b(21) : Gain  Gain=0.317166497217694909  ParamDataTypeStr=double  RndMeth=Nearest  SaturateOnIntegerOverflow=on  OutDataTypeStr=Inherit: Same as input
  b(22) : Gain  Gain=0.485387646787325211  ParamDataTypeStr=double  RndMeth=Nearest  SaturateOnIntegerOverflow=on  OutDataTypeStr=Inherit: Same as input
  b(23) : Gain  Gain=0.317166497217694909  ParamDataTypeStr=double  RndMeth=Nearest  SaturateOnIntegerOverflow=on  OutDataTypeStr=Inherit: Same as input
  b(24) : Gain  Gain=0.0144622757712384552  ParamDataTypeStr=double  RndMeth=Nearest  SaturateOnIntegerOverflow=on  OutDataTypeStr=Inherit: Same as input
  b(25) : Gain  Gain=-0.102724668578821676  ParamDataTypeStr=double  RndMeth=Nearest  SaturateOnIntegerOverflow=on  OutDataTypeStr=Inherit: Same as input
  b(26) : Gain  Gain=-0.0140480435158088935  ParamDataTypeStr=double  RndMeth=Nearest  SaturateOnIntegerOverflow=on  OutDataTypeStr=Inherit: Same as input
  b(27) : Gain  Gain=0.0581554658147298703  ParamDataTypeStr=double  RndMeth=Nearest  SaturateOnIntegerOverflow=on  OutDataTypeStr=Inherit: Same as input
  b(28) : Gain  Gain=0.0133889451993669008  ParamDataTypeStr=double  RndMeth=Nearest  SaturateOnIntegerOverflow=on  OutDataTypeStr=Inherit: Same as input
  b(29) : Gain  Gain=-0.0379966231454636413  ParamDataTypeStr=double  RndMeth=Nearest  SaturateOnIntegerOverflow=on  OutDataTypeStr=Inherit: Same as input
  b(3) : Gain  Gain=0.00677034464011870129  ParamDataTypeStr=double  RndMeth=Nearest  SaturateOnIntegerOverflow=on  OutDataTypeStr=Inherit: Same as input
  b(30) : Gain  Gain=-0.0124890278353230171  ParamDataTypeStr=double  RndMeth=Nearest  SaturateOnIntegerOverflow=on  OutDataTypeStr=Inherit: Same as input
  b(31) : Gain  Gain=0.026175888580407581  ParamDataTypeStr=double  RndMeth=Nearest  SaturateOnIntegerOverflow=on  OutDataTypeStr=Inherit: Same as input
  b(32) : Gain  Gain=0.0114319620717779676  ParamDataTypeStr=double  RndMeth=Nearest  SaturateOnIntegerOverflow=on  OutDataTypeStr=Inherit: Same as input
  b(33) : Gain  Gain=-0.0182735187337824609  ParamDataTypeStr=double  RndMeth=Nearest  SaturateOnIntegerOverflow=on  OutDataTypeStr=Inherit: Same as input
  b(34) : Gain  Gain=-0.0101212347032790025  ParamDataTypeStr=double  RndMeth=Nearest  SaturateOnIntegerOverflow=on  OutDataTypeStr=Inherit: Same as input
  b(35) : Gain  Gain=0.0129828838088557105  ParamDataTypeStr=double  RndMeth=Nearest  SaturateOnIntegerOverflow=on  OutDataTypeStr=Inherit: Same as input
  b(36) : Gain  Gain=0.00925679761513798632  ParamDataTypeStr=double  RndMeth=Nearest  SaturateOnIntegerOverflow=on  OutDataTypeStr=Inherit: Same as input
  b(37) : Gain  Gain=-0.00840161718602687457  ParamDataTypeStr=double  RndMeth=Nearest  SaturateOnIntegerOverflow=on  OutDataTypeStr=Inherit: Same as input
  b(38) : Gain  Gain=-0.00623114541414451859  ParamDataTypeStr=double  RndMeth=Nearest  SaturateOnIntegerOverflow=on  OutDataTypeStr=Inherit: Same as input
  b(39) : Gain  Gain=0.0111170760810775926  ParamDataTypeStr=double  RndMeth=Nearest  SaturateOnIntegerOverflow=on  OutDataTypeStr=Inherit: Same as input
  b(4) : Gain  Gain=0.016731945423489044  ParamDataTypeStr=double  RndMeth=Nearest  SaturateOnIntegerOverflow=on  OutDataTypeStr=Inherit: Same as input
  b(40) : Gain  Gain=0.016731945423489044  ParamDataTypeStr=double  RndMeth=Nearest  SaturateOnIntegerOverflow=on  OutDataTypeStr=Inherit: Same as input
  b(41) : Gain  Gain=0.00677034464011870129  ParamDataTypeStr=double  RndMeth=Nearest  SaturateOnIntegerOverflow=on  OutDataTypeStr=Inherit: Same as input
  b(42) : Gain  Gain=-0.00208324498207925878  ParamDataTypeStr=double  RndMeth=Nearest  SaturateOnIntegerOverflow=on  OutDataTypeStr=Inherit: Same as input
  b(43) : Gain  Gain=-0.00242287385232693503  ParamDataTypeStr=double  RndMeth=Nearest  SaturateOnIntegerOverflow=on  OutDataTypeStr=Inherit: Same as input
  b(5) : Gain  Gain=0.0111170760810775926  ParamDataTypeStr=double  RndMeth=Nearest  SaturateOnIntegerOverflow=on  OutDataTypeStr=Inherit: Same as input
  b(6) : Gain  Gain=-0.00623114541414451859  ParamDataTypeStr=double  RndMeth=Nearest  SaturateOnIntegerOverflow=on  OutDataTypeStr=Inherit: Same as input
  b(7) : Gain  Gain=-0.00840161718602687457  ParamDataTypeStr=double  RndMeth=Nearest  SaturateOnIntegerOverflow=on  OutDataTypeStr=Inherit: Same as input
  b(8) : Gain  Gain=0.00925679761513798632  ParamDataTypeStr=double  RndMeth=Nearest  SaturateOnIntegerOverflow=on  OutDataTypeStr=Inherit: Same as input
  b(9) : Gain  Gain=0.0129828838088557105  ParamDataTypeStr=double  RndMeth=Nearest  SaturateOnIntegerOverflow=on  OutDataTypeStr=Inherit: Same as input
  Output : Outport
  wires:
  Input/1 -> b(1)/1, BodyDelay2/1
  b(1)/1 -> BodyLSum2/2
  BodyDelay2/1 -> b(2)/1, BodyDelay3/1
  b(2)/1 -> BodyLSum2/1
  BodyLSum2/1 -> BodyLSum3/2
  BodyDelay3/1 -> b(3)/1, BodyDelay4/1
  b(3)/1 -> BodyLSum3/1
  BodyLSum3/1 -> BodyLSum4/2
  BodyDelay4/1 -> b(4)/1, BodyDelay5/1
  b(4)/1 -> BodyLSum4/1
  BodyLSum4/1 -> BodyLSum5/2
  BodyDelay5/1 -> b(5)/1, BodyDelay6/1
  b(5)/1 -> BodyLSum5/1
  BodyLSum5/1 -> BodyLSum6/2
  BodyDelay6/1 -> b(6)/1, BodyDelay7/1
  b(6)/1 -> BodyLSum6/1
  BodyLSum6/1 -> BodyLSum7/2
  BodyDelay7/1 -> b(7)/1, BodyDelay8/1
  b(7)/1 -> BodyLSum7/1
  BodyLSum7/1 -> BodyLSum8/2
  BodyDelay8/1 -> b(8)/1, BodyDelay9/1
  b(8)/1 -> BodyLSum8/1
  BodyLSum8/1 -> BodyLSum9/2
  BodyDelay9/1 -> b(9)/1, BodyDelay10/1
  b(9)/1 -> BodyLSum9/1
  BodyLSum9/1 -> BodyLSum10/2
  BodyDelay10/1 -> b(10)/1, BodyDelay11/1
  b(10)/1 -> BodyLSum10/1
  BodyLSum10/1 -> BodyLSum11/2
  BodyDelay11/1 -> b(11)/1, BodyDelay12/1
  b(11)/1 -> BodyLSum11/1
  BodyLSum11/1 -> BodyLSum12/2
  BodyDelay12/1 -> b(12)/1, BodyDelay13/1
  b(12)/1 -> BodyLSum12/1
  BodyLSum12/1 -> BodyLSum13/2
  BodyDelay13/1 -> b(13)/1, BodyDelay14/1
  b(13)/1 -> BodyLSum13/1
  BodyLSum13/1 -> BodyLSum14/2
  BodyDelay14/1 -> b(14)/1, BodyDelay15/1
  b(14)/1 -> BodyLSum14/1
  BodyLSum14/1 -> BodyLSum15/2
  BodyDelay15/1 -> b(15)/1, BodyDelay16/1
  b(15)/1 -> BodyLSum15/1
  BodyLSum15/1 -> BodyLSum16/2
  BodyDelay16/1 -> b(16)/1, BodyDelay17/1
  b(16)/1 -> BodyLSum16/1
  BodyLSum16/1 -> BodyLSum17/2
  BodyDelay17/1 -> b(17)/1, BodyDelay18/1
  b(17)/1 -> BodyLSum17/1
  BodyLSum17/1 -> BodyLSum18/2
  BodyDelay18/1 -> b(18)/1, BodyDelay19/1
  b(18)/1 -> BodyLSum18/1
  BodyLSum18/1 -> BodyLSum19/2
  BodyDelay19/1 -> b(19)/1, BodyDelay20/1
  b(19)/1 -> BodyLSum19/1
  BodyLSum19/1 -> BodyLSum20/2
  BodyDelay20/1 -> b(20)/1, BodyDelay21/1
  b(20)/1 -> BodyLSum20/1
  BodyLSum20/1 -> BodyLSum21/2
  BodyDelay21/1 -> b(21)/1, BodyDelay22/1
  b(21)/1 -> BodyLSum21/1
  BodyLSum21/1 -> BodyLSum22/2
  BodyDelay22/1 -> b(22)/1, BodyDelay23/1
  b(22)/1 -> BodyLSum22/1
  BodyLSum22/1 -> BodyLSum23/2
  BodyDelay23/1 -> b(23)/1, BodyDelay24/1
  b(23)/1 -> BodyLSum23/1
  BodyLSum23/1 -> BodyLSum24/2
  BodyDelay24/1 -> b(24)/1, BodyDelay25/1
  b(24)/1 -> BodyLSum24/1
  BodyLSum24/1 -> BodyLSum25/2
  BodyDelay25/1 -> b(25)/1, BodyDelay26/1
  b(25)/1 -> BodyLSum25/1
  BodyLSum25/1 -> BodyLSum26/2
  BodyDelay26/1 -> b(26)/1, BodyDelay27/1
  b(26)/1 -> BodyLSum26/1
  BodyLSum26/1 -> BodyLSum27/2
  BodyDelay27/1 -> b(27)/1, BodyDelay28/1
  b(27)/1 -> BodyLSum27/1
  BodyLSum27/1 -> BodyLSum28/2
  BodyDelay28/1 -> b(28)/1, BodyDelay29/1
  b(28)/1 -> BodyLSum28/1
  BodyLSum28/1 -> BodyLSum29/2
  BodyDelay29/1 -> b(29)/1, BodyDelay30/1
  b(29)/1 -> BodyLSum29/1
  BodyLSum29/1 -> BodyLSum30/2
  BodyDelay30/1 -> b(30)/1, BodyDelay31/1
  b(30)/1 -> BodyLSum30/1
  BodyLSum30/1 -> BodyLSum31/2
  BodyDelay31/1 -> b(31)/1, BodyDelay32/1
  b(31)/1 -> BodyLSum31/1
  BodyLSum31/1 -> BodyLSum32/2
  BodyDelay32/1 -> b(32)/1, BodyDelay33/1
  b(32)/1 -> BodyLSum32/1
  BodyLSum32/1 -> BodyLSum33/2
  BodyDelay33/1 -> b(33)/1, BodyDelay34/1
  b(33)/1 -> BodyLSum33/1
  BodyLSum33/1 -> BodyLSum34/2
  BodyDelay34/1 -> b(34)/1, BodyDelay35/1
  b(34)/1 -> BodyLSum34/1
  BodyLSum34/1 -> BodyLSum35/2
  BodyDelay35/1 -> b(35)/1, BodyDelay36/1
  b(35)/1 -> BodyLSum35/1
  BodyLSum35/1 -> BodyLSum36/2
  BodyDelay36/1 -> b(36)/1, BodyDelay37/1
  b(36)/1 -> BodyLSum36/1
  BodyLSum36/1 -> BodyLSum37/2
  BodyDelay37/1 -> b(37)/1, BodyDelay38/1
  b(37)/1 -> BodyLSum37/1
  BodyLSum37/1 -> BodyLSum38/2
  BodyDelay38/1 -> b(38)/1, BodyDelay39/1
  b(38)/1 -> BodyLSum38/1
  BodyLSum38/1 -> BodyLSum39/2
  BodyDelay39/1 -> b(39)/1, BodyDelay40/1
  b(39)/1 -> BodyLSum39/1
  BodyLSum39/1 -> BodyLSum40/2
  BodyDelay40/1 -> b(40)/1, BodyDelay41/1
  b(40)/1 -> BodyLSum40/1
  BodyLSum40/1 -> BodyLSum41/2
  BodyDelay41/1 -> b(41)/1, BodyDelay42/1
  b(41)/1 -> BodyLSum41/1
  BodyLSum41/1 -> BodyLSum42/2
  BodyDelay42/1 -> b(42)/1, BodyDelay43/1
  b(42)/1 -> BodyLSum42/1
  BodyLSum42/1 -> BodyLSum43/1
  BodyDelay43/1 -> b(43)/1
  b(43)/1 -> BodyLSum43/2
  BodyLSum43/1 -> Output/1
